simulink model "mconversion2"  (Simulink 8.0)
settings: Solver=ode3  StartTime=0.0  StopTime=10.0  RelTol=1e-3
settings Model: Creator=awarlock  LastModifiedBy=htu  ExtModeAutoUpdateStatusClock=off
settings DataIOCC: SignalLoggingSaveFormat=ModelDataLogs  SignalLoggingName=logsOut
settings OptimizationCC: InlineParams=on  InlineInvariantSignals=on  InitFltsAndDblsToZero=on  LifeSpan=1
settings DebuggingCC: SaveWithParameterizedLinksMsg=none  SolverPrmCheckMsg=none  MultiTaskDSMMsg=warning  MultiTaskCondExecSysMsg=none
settings HardwareCC: ProdHWDeviceType=Specified
settings RTWCC: SystemTargetFile=ert.tlc  TemplateMakefile=ert_default_tmf  Description=RTW Embedded Coder  ProcessScript=ert_make_rtw_hook  IncludeERTFirstTime=on
settings CodeAppCC: IgnoreCustomStorageClasses=off
settings ERTTargetCC: TargetFcnLib=iso_c_tmw.mat  CodeReplacementLibrary=ANSI_C  MultiwordLength=2048  GenerateSampleERTMain=on  ERTCustomFileTemplate=example_file_process.tlc  ConvertIfToSwitch=off  SuppressUnreachableDefaultCases=off

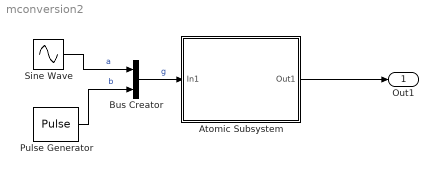
== system mconversion2 ==
  Atomic Subsystem : Subsystem  TreatAsAtomicUnit=on
  Bus Creator : BusCreator  Inputs=2
  Pulse Generator : DiscretePulseGenerator  SampleTime=0.1
  Sine Wave : Sin  SampleTime=0.1
  Out1 : Outport
  wires:
  Sine Wave/1 -> Bus Creator/1  "a"
  Pulse Generator/1 -> Bus Creator/2  "b"
  Bus Creator/1 -> Atomic Subsystem/1(In1)  "g"
  Atomic Subsystem/1(Out1) -> Out1/1

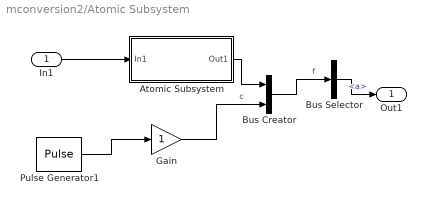
== system mconversion2/Atomic Subsystem ==
  In1 : Inport
  Atomic Subsystem : Subsystem  TreatAsAtomicUnit=on
  Bus Creator : BusCreator  Inputs=2
  Bus Selector : BusSelector  OutputSignals=e.g.a
  Gain : Gain
  Pulse Generator1 : DiscretePulseGenerator  SampleTime=0.1
  Out1 : Outport
  wires:
  In1/1 -> Atomic Subsystem/1(In1)
  Pulse Generator1/1 -> Gain/1
  Gain/1 -> Bus Creator/2  "c"
  Atomic Subsystem/1(Out1) -> Bus Creator/1
  Bus Creator/1 -> Bus Selector/1  "f"
  Bus Selector/1 -> Out1/1  "<a>"

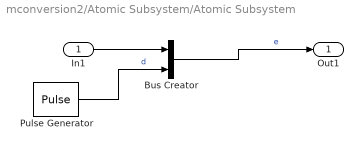
== system mconversion2/Atomic Subsystem/Atomic Subsystem ==
  In1 : Inport
  Bus Creator : BusCreator  Inputs=2
  Pulse Generator : DiscretePulseGenerator  SampleTime=0.1
  Out1 : Outport
  wires:
  In1/1 -> Bus Creator/1
  Pulse Generator/1 -> Bus Creator/2  "d"
  Bus Creator/1 -> Out1/1  "e"
